simulink model "px4demo_attitude_system_hil"  (R2016b)
settings: Solver=FixedStepAuto  StartTime=0.0  StopTime=inf  RelTol=1e-3
PostLoadFcn:
  | kFactor = 1.2;
  | 
  | KpRollAttitude = 0.630138625117681 / kFactor;
  | KiRollAttitude = 0.0552303199591522 / kFactor;
  | 
  | KpPitchAttitude = 0.630138625117681 / kFactor;
  | KiPitchAttitude = 0.0552303199591522 / kFactor;
  | 
  | KpRollRate = 1.31533836563383 / kFactor;
  | KiRollRate = 0.460338699849681 / kFactor;
  | 
  | KpPitchRate = 1.31533836563383 / kFactor;
  | KiPitchRate = 0.460338699849681 / kFactor;
  | 
  | KpYawRate = 1.31533836563383 / kFactor;
  | KiYawRate = 0.460338699849681 / kFactor;
undefined symbols (not defined in the file or in its folder): PX4_TUNE_ENUM, RGBLED_COLOR_ENUM, RGBLED_MODE_ENUM
libraries: pixhawk_slib_sensors_actuators x4, pixhawk_slib_ADC_serial x2
settings Model: Creator=Steve  LastModifiedBy=E6320
settings SolverCC: AutoInsertRateTranBlk=on
settings DataIOCC: LimitDataPoints=on  SaveFormat=Array
settings OptimizationCC: DefaultParameterBehavior=Inlined  LifeSpan=1  MaxStackSize=64
settings DebuggingCC: SolverPrmCheckMsg=warning  AllowSymbolicDim=off  SFUnexpectedBacktrackingDiag=warning  SFNoUnconditionalDefaultTransitionDiag=warning  SFExecutionAtInitializationDiag=none
settings HardwareCC: ProdBitPerPointer=32  ProdBitPerSizeT=32  ProdBitPerPtrDiffT=32  ProdLargestAtomicInteger=Long  ProdLargestAtomicFloat=Double  ProdWordSize=32  ProdHWDeviceType=ARM Compatible->ARM Cortex
settings ModelReferenceCC: PropagateSignalLabelsOutOfModel=off
settings RTWCC: SystemTargetFile=ert.tlc  HardwareBoard=Pixhawk PX4  TemplateMakefile=ert_default_tmf  Description=Embedded Coder  GenerateReport=on  Toolchain=Pixhawk Toolchain  IncludeHyperlinkInReport=on  LaunchReport=on  GenerateTraceReport=on  GenerateTraceReportSl=on  GenerateTraceReportSf=on  GenerateTraceReportEml=on  GenerateCodeMetricsReport=on
settings CodeAppCC: IgnoreCustomStorageClasses=off
settings ERTTargetCC: CodeReplacementLibrary=GCC ARM Cortex-A9  ExtModeTransport=1  ExtModeMexFile=ext_serial_win32_comm  ExtModeMexArgs=/dev/serial  ERTCustomFileTemplate=PX4_codertarget_file_process.tlc  ConvertIfToSwitch=off  SuppressUnreachableDefaultCases=off
settings ConfigComp: CovMetricSettings=dw  CovHtmlReporting=on  CovSaveCumulativeToWorkspaceVar=on  CovSaveSingleToWorkspaceVar=on  CovExternalEMLEnable=off  CovSFcnEnable=off

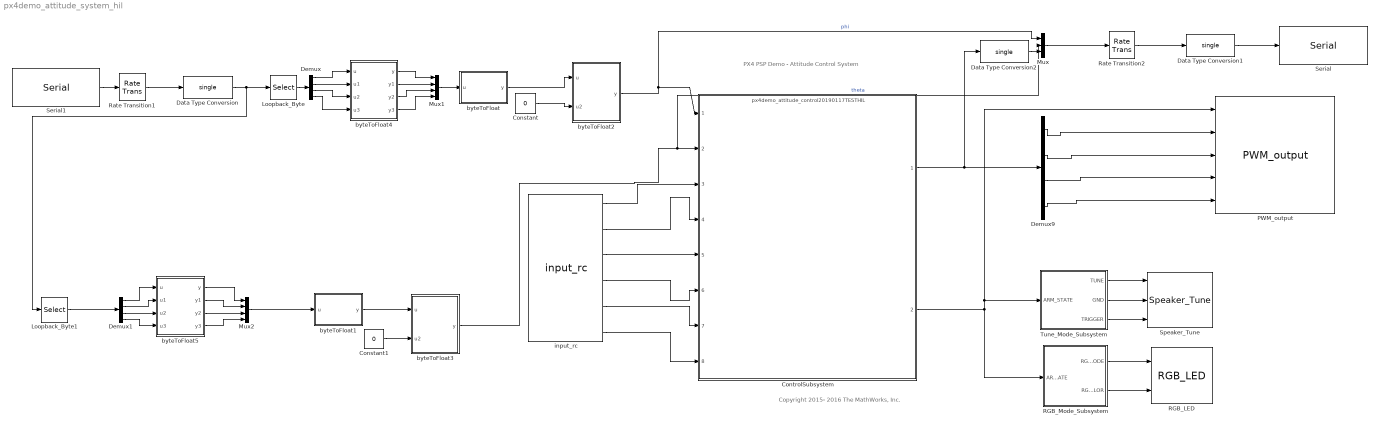
== system px4demo_attitude_system_hil ==
  note: PX4 PSP Demo - Attitude Control System
  note: Copyright 2015- 2016 The MathWorks, Inc.
  Constant : Constant  Value=0  OutDataTypeStr=single
  Constant1 : Constant  Value=0  OutDataTypeStr=single
  ControlSubsystem : ModelReference  ModelNameDialog=px4demo_attitude_control20190117TESTHIL.slx  SimulationMode=Normal  ModelReferenceVersion=1.297
  Data Type Conversion : DataTypeConversion  OutDataTypeStr=single
  Data Type Conversion1 : DataTypeConversion  OutDataTypeStr=single
  Data Type Conversion2 : DataTypeConversion  OutDataTypeStr=single
  Demux : Demux
  Demux1 : Demux
  Demux9 : Demux
  Loopback_Byte : Selector  InputPortWidth=8  IndexOptions=Index vector (dialog)  Indices=1:4  OutputSizes=1
  Loopback_Byte1 : Selector  InputPortWidth=8  IndexOptions=Index vector (dialog)  Indices=5:8  OutputSizes=1
  Mux : Mux  Inputs=3
  Mux1 : Mux
  Mux2 : Mux
  PWM_output : pixhawk_slib_sensors_actuators/PWM_output  pwm_rate=50Hz  show_pwm1=on  show_pwm2=on  show_pwm3=on  show_pwm4=on  show_pwm5=off  show_pwm6=off  show_pwm7=off  show_pwm8=off
  RGB_LED : pixhawk_slib_sensors_actuators/RGB_LED
  RGB_Mode_Subsystem : Subsystem
  Rate Transition1 : RateTransition  OutPortSampleTimeMultiple=1.5  OutPortSampleTime=0.3
  Rate Transition2 : RateTransition  Integrity=off  Deterministic=off  OutPortSampleTimeMultiple=1.5  OutPortSampleTime=1.5
  Serial : pixhawk_slib_ADC_serial/Serial  DeviceName=/dev/ttyS1  ReadOrWrite=Writing  BaudRateStr=57600  block=off  WriteStatus=on  Terminator=off  Header=off  NumBytesRead=4  TerminatorChar=\n  HeaderData=57600  SimulateUsing=Code generation
  Serial1 : pixhawk_slib_ADC_serial/Serial  DeviceName=/dev/ttyS1  ReadOrWrite=Reading  BaudRateStr=57600  block=off  WriteStatus=off  Terminator=off  Header=off  NumBytesRead=8  TerminatorChar=\n  HeaderData=57600  SimulateUsing=Code generation
  Speaker_Tune : pixhawk_slib_sensors_actuators/Speaker_Tune
  Tune_Mode_Subsystem : Subsystem
  byteToFloat : MATLAB Function  TreatAsAtomicUnit=on
  byteToFloat1 : MATLAB Function  TreatAsAtomicUnit=on
  byteToFloat2 : MATLAB Function  TreatAsAtomicUnit=on
  byteToFloat3 : MATLAB Function  TreatAsAtomicUnit=on
  byteToFloat4 : MATLAB Function  TreatAsAtomicUnit=on
  byteToFloat5 : MATLAB Function  TreatAsAtomicUnit=on
  input_rc : pixhawk_slib_sensors_actuators/input_rc  sampletime=1/250  channel1=on  channel2=on  channel3=on  channel4=on  channel5=on  channel6=on  channel7=off  channel8=off  ch_count=off  rssi=off  rc_failsafe=off  rc_lost=off  rc_inputsource=off
  wires:
  Demux9/4 -> PWM_output/5
  Demux9/2 -> PWM_output/3
  Demux9/3 -> PWM_output/4
  Demux9/1 -> PWM_output/2
  RGB_Mode_Subsystem/1(RGB_MODE) -> RGB_LED/1
  RGB_Mode_Subsystem/2(RGB_COLOR) -> RGB_LED/2
  Tune_Mode_Subsystem/1(TUNE) -> Speaker_Tune/1
  Tune_Mode_Subsystem/2(GND) -> Speaker_Tune/2
  Tune_Mode_Subsystem/3(TRIGGER) -> Speaker_Tune/3
  ControlSubsystem/2 -> RGB_Mode_Subsystem/1(ARM_STATE), Tune_Mode_Subsystem/1(ARM_STATE), PWM_output/1
  byteToFloat2/1(y) -> Mux/1, ControlSubsystem/1  "phi"
  byteToFloat3/1(y) -> Mux/2, ControlSubsystem/2  "theta"
  input_rc/1 -> ControlSubsystem/3
  input_rc/2 -> ControlSubsystem/4
  input_rc/3 -> ControlSubsystem/5
  input_rc/4 -> ControlSubsystem/6
  input_rc/5 -> ControlSubsystem/7
  ControlSubsystem/1 -> Demux9/1, Data Type Conversion2/1
  input_rc/6 -> ControlSubsystem/8
  Serial1/1 -> Rate Transition1/1
  byteToFloat/1(y) -> byteToFloat2/1(u)
  Data Type Conversion1/1 -> Serial/1
  Rate Transition2/1 -> Data Type Conversion1/1
  byteToFloat1/1(y) -> byteToFloat3/1(u)
  Mux/1 -> Rate Transition2/1
  Data Type Conversion2/1 -> Mux/3
  Rate Transition1/1 -> Data Type Conversion/1
  Constant/1 -> byteToFloat2/2(u2)
  Constant1/1 -> byteToFloat3/2(u2)
  Data Type Conversion/1 -> Loopback_Byte/1, Loopback_Byte1/1
  Loopback_Byte/1 -> Demux/1
  Mux1/1 -> byteToFloat/1(u)
  Mux2/1 -> byteToFloat1/1(u)
  Loopback_Byte1/1 -> Demux1/1
  Demux/1 -> byteToFloat4/1(u)
  Demux/2 -> byteToFloat4/2(u1)
  Demux/3 -> byteToFloat4/3(u2)
  Demux/4 -> byteToFloat4/4(u3)
  byteToFloat4/4(y3) -> Mux1/4
  byteToFloat4/3(y2) -> Mux1/3
  byteToFloat4/2(y1) -> Mux1/2
  byteToFloat4/1(y) -> Mux1/1
  Demux1/1 -> byteToFloat5/1(u)
  Demux1/2 -> byteToFloat5/2(u1)
  Demux1/3 -> byteToFloat5/3(u2)
  Demux1/4 -> byteToFloat5/4(u3)
  byteToFloat5/4(y3) -> Mux2/4
  byteToFloat5/3(y2) -> Mux2/3
  byteToFloat5/2(y1) -> Mux2/2
  byteToFloat5/1(y) -> Mux2/1

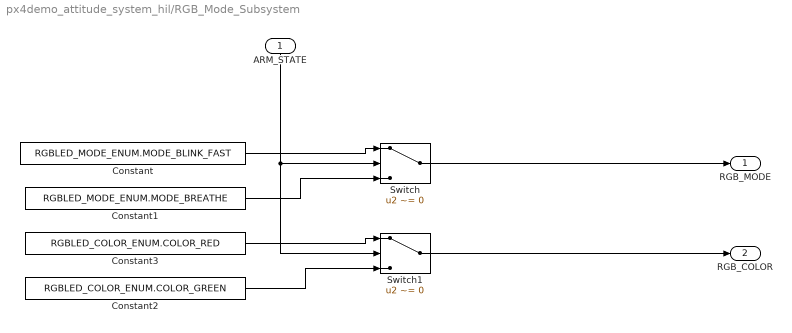
== system px4demo_attitude_system_hil/RGB_Mode_Subsystem ==
  ARM_STATE : Inport
  Constant : Constant  Value=RGBLED_MODE_ENUM.MODE_BLINK_FAST  OutDataTypeStr=Enum: RGBLED_MODE_ENUM
  Constant1 : Constant  Value=RGBLED_MODE_ENUM.MODE_BREATHE  OutDataTypeStr=Enum: RGBLED_MODE_ENUM
  Constant2 : Constant  Value=RGBLED_COLOR_ENUM.COLOR_GREEN  OutDataTypeStr=Enum: RGBLED_COLOR_ENUM
  Constant3 : Constant  Value=RGBLED_COLOR_ENUM.COLOR_RED  OutDataTypeStr=Enum: RGBLED_COLOR_ENUM
  Switch : Switch  Criteria=u2 ~= 0  Threshold=1500  SampleTime=1/2
  Switch1 : Switch  Criteria=u2 ~= 0  Threshold=1500  SampleTime=1/2
  RGB_MODE : Outport
  RGB_COLOR : Outport  Port=2
  wires:
  ARM_STATE/1 -> Switch1/2, Switch/2
  Constant/1 -> Switch/1
  Constant1/1 -> Switch/3
  Switch/1 -> RGB_MODE/1
  Constant3/1 -> Switch1/1
  Constant2/1 -> Switch1/3
  Switch1/1 -> RGB_COLOR/1

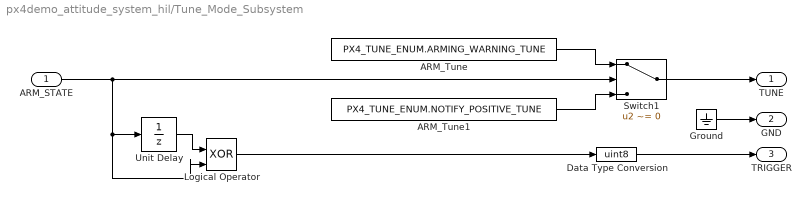
== system px4demo_attitude_system_hil/Tune_Mode_Subsystem ==
  ARM_STATE : Inport
  ARM_Tune : Constant  Value=PX4_TUNE_ENUM.ARMING_WARNING_TUNE  OutDataTypeStr=Enum: PX4_TUNE_ENUM
  ARM_Tune1 : Constant  Value=PX4_TUNE_ENUM.NOTIFY_POSITIVE_TUNE  OutDataTypeStr=Enum: PX4_TUNE_ENUM
  Data Type Conversion : DataTypeConversion  OutDataTypeStr=uint8
  Ground : Ground
  Logical Operator : Logic  Operator=XOR  IconShape=distinctive  AllPortsSameDT=off  OutDataTypeStr=boolean
  Switch1 : Switch  Criteria=u2 ~= 0  Threshold=1500
  Unit Delay : UnitDelay  SampleTime=-1
  TUNE : Outport
  GND : Outport  Port=2
  TRIGGER : Outport  Port=3
  wires:
  Ground/1 -> GND/1
  Data Type Conversion/1 -> TRIGGER/1
  Switch1/1 -> TUNE/1
  ARM_Tune/1 -> Switch1/1
  ARM_Tune1/1 -> Switch1/3
  ARM_STATE/1 -> Logical Operator/2, Unit Delay/1, Switch1/2
  Unit Delay/1 -> Logical Operator/1
  Logical Operator/1 -> Data Type Conversion/1

== matlab function px4demo_attitude_system_hil/byteToFloat1 ==
  data: u input; y output
function y = fcn(u)
%#codegen
y = single(0);
y = single(typecast(uint8(u),'single'));
% y = u;

== matlab function px4demo_attitude_system_hil/byteToFloat2 ==
  data: u input; y output; u2 input
function y = fcn(u,u2)
u1=abs(u);
if(u1>=10)
    y=u2;
elseif(u1<=0.00001)
    y=u2;
else
    y=u;
end

== matlab function px4demo_attitude_system_hil/byteToFloat3 ==
  data: u input; y output; u2 input
function y = fcn(u,u2)
u1=abs(u);
if(u1>=10)
    y=u2;
elseif(u1<=0.00001)
    y=u2;
else
    y=u;
end

== matlab function px4demo_attitude_system_hil/byteToFloat4 ==
  data: u input; y output; u1 input; y1 output; u2 input; u3 input; y2 output; y3 output
function [y,y1,y2,y3]= fcn(u,u1,u2,u3)
if(u2 >= 128 && u3==255)
    y=single(0);
    y1=single(0);
    y2=single(0);
    y3=single(0);
else
    y=single(u);
    y1=single(u1);
    y2=single(u2);
    y3=single(u3);
end

== matlab function px4demo_attitude_system_hil/byteToFloat5 ==
  data: u input; y output; u1 input; y1 output; u2 input; u3 input; y2 output; y3 output
function [y,y1,y2,y3]= fcn(u,u1,u2,u3)
if(u2 >= 128 && u3==255)
    y=single(0);
    y1=single(0);
    y2=single(0);
    y3=single(0);
else
    y=single(u);
    y1=single(u1);
    y2=single(u2);
    y3=single(u3);
end

== matlab function px4demo_attitude_system_hil/byteToFloat ==
  data: u input; y output
function y = fcn(u)
%#codegen
y = single(0);
y = single(typecast(uint8(u),'single'));
% y = u;
